simulink model "rpi_motor_cal"  (R2022b)
settings: Solver=FixedStepAuto  StartTime=0.0  StopTime=2  RelTol=1e-3  EnableMultiTasking=on
undefined symbols (not defined in the file or in its folder): A, b
libraries: raspberrypiBasiclib x6, robotmobilelib x1, raspberrypiIMUsensorslib x1, dspsigops x1
settings Model: Creator=sjohnson  LastModifiedBy=sjohnson
settings SolverCC: PositivePriorityOrder=on
settings OptimizationCC: EnhancedBackFolding=on  PassReuseOutputArgsAs=Individual arguments  ZeroExternalMemoryAtStartup=off  ZeroInternalMemoryAtStartup=off  MaxStackSize=64  OptimizeBlockOrder=speed  DifferentSizesBufferReuse=on  OptimizationCustomize=off  EfficientTunableParamExpr=on
settings DebuggingCC: ParameterTunabilityLossMsg=error
settings HardwareCC: ProdBitPerPointer=32  ProdBitPerSizeT=32  ProdBitPerPtrDiffT=32  ProdLargestAtomicInteger=Long  ProdLargestAtomicFloat=Double  ProdWordSize=32  ProdLongLongMode=on  ProdHWDeviceType=ARM Compatible->ARM Cortex  UseEmbeddedCoderFeatures=off  UseSimulinkCoderFeatures=off
settings RTWCC: Description=Embedded Coder  SystemTargetFile=ert.tlc  HardwareBoard=Raspberry Pi  TLCOptions="-aInlineSetEventsForThisBaseRateFcn=TLC_FALSE -aSuppressMultiTaskScheduler=TLC_FALSE  -aRateBasedStepFcn=0"  TemplateMakefile=ert_default_tmf  Toolchain=GNU GCC Embedded Linux  BuildConfiguration=Faster Runs
settings CodeAppCC: ForceParamTrailComments=on  IgnoreCustomStorageClasses=off  OperatorAnnotations=on  SimulinkDataObjDesc=on  SFDataObjDesc=on  InsertBlockDesc=on
settings ERTTargetCC: SupportNonInlinedSFcns=on  SupportVariableSizeSignals=on  ExtModeTransport=2  ExtModeStaticAlloc=on  ExtModeMexFile=ext_xcp  ExtModeIntrfLevel=Level2 - Open

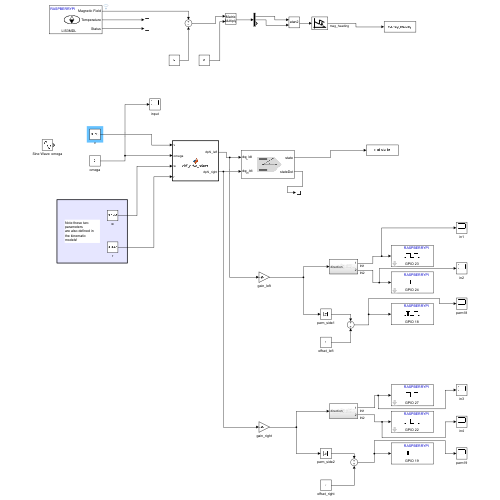
[thumbnail: Simulink's stored preview of the top-level diagram]
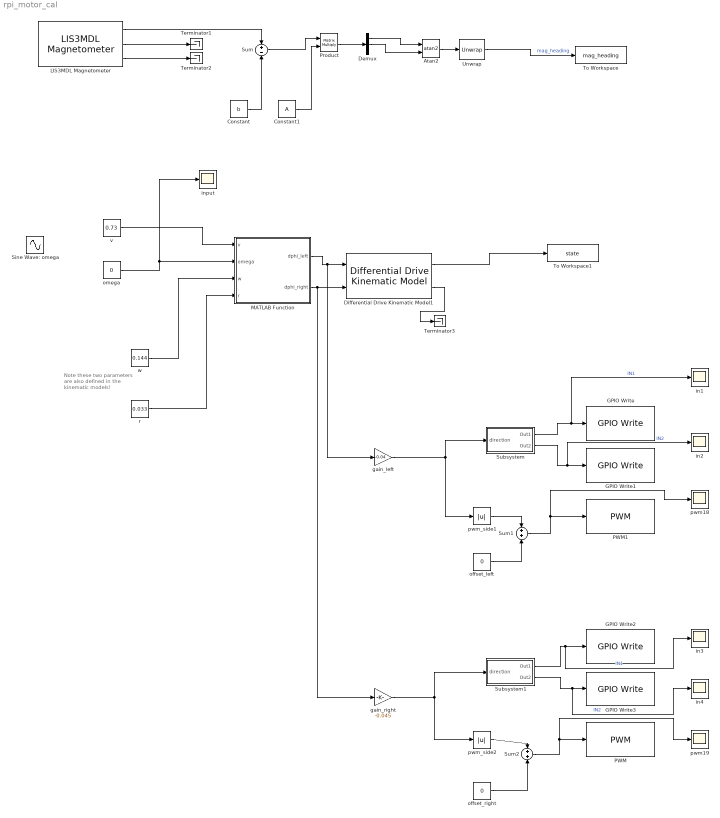
== system rpi_motor_cal ==
  note: Note these two parameters
      | are also defined in the kinematic
      | models!
  Atan2 : Trigonometry  Operator=atan2
  Constant : Constant  Value=b
  Constant1 : Constant  Value=A
  Demux : Demux  Outputs=3
  Differential Drive Kinematic Model1 : robotmobilelib/Differential Drive Kinematic Model  VehicleInputs=Wheel Speeds  WheelRadius=.033  WheelSpeedRange=[-inf inf]  TrackWidth=0.144  InitialState=[0; 0; 0]  SimulateUsing=Interpreted execution
  GPIO Write : raspberrypiBasiclib/GPIO Write  board=Pi 4 Model B  gpio=23  direction=Output  blockPlatform=Raspberry Pi
  GPIO Write1 : raspberrypiBasiclib/GPIO Write  board=Pi 4 Model B  gpio=24  direction=Output  blockPlatform=Raspberry Pi
  GPIO Write2 : raspberrypiBasiclib/GPIO Write  board=Pi 4 Model B  gpio=27  direction=Output  blockPlatform=Raspberry Pi
  GPIO Write3 : raspberrypiBasiclib/GPIO Write  board=Pi 4 Model B  gpio=22  direction=Output  blockPlatform=Raspberry Pi
  LIS3MDL Magnetometer : raspberrypiIMUsensorslib/LIS3MDL Magnetometer  I2CModule=1  I2CAddress=0x1E  IsActiveMagnetometer=on  IsActiveTemperature=on  IsStatus=on  SampleTime=-1  MagnetometerRange=+/- 400 uT  MagnetometerODR=40 Hz
  MATLAB Function : MATLAB Function  TreatAsAtomicUnit=on
  PWM : raspberrypiBasiclib/PWM  board=Pi 4 Model B  Pin_=19  Frequency=50  blockPlatform=Raspberry Pi
  PWM1 : raspberrypiBasiclib/PWM  board=Pi 4 Model B  Pin_=18  Frequency=50  blockPlatform=Raspberry Pi
  Product : Product  Multiplication=Matrix(*)
  Sine Wave: omega : Sin  Amplitude=0.1  Frequency=0.1  SampleTime=0
  Subsystem : Subsystem
  Subsystem1 : Subsystem
  Sum : Sum  Inputs=+-
  Sum1 : Sum
  Sum2 : Sum
  Terminator1 : Terminator
  Terminator2 : Terminator
  Terminator3 : Terminator
  To Workspace : ToWorkspace  VariableName=mag_heading  SaveFormat=Structure With Time  SampleTime=-1
  To Workspace1 : ToWorkspace  VariableName=state  SaveFormat=Structure With Time  SampleTime=-1
  Unwrap : dspsigops/Unwrap  tol=pi  InputProcessing=Columns as channels (frame based)  running=off
  gain_left : Gain  Gain=-0.04
  gain_right : Gain  Gain=-0.045
  in{1..4} (4 alike) : Scope
  input : Scope
  offset_left : Constant  Value=0
  offset_right : Constant  Value=0
  omega : Constant  Value=0
  pwm18 : Scope
  pwm19 : Scope
  pwm_side1 : Abs  SaturateOnIntegerOverflow=off
  pwm_side2 : Abs  SaturateOnIntegerOverflow=off
  r : Constant  Value=0.033
  v : Constant  Value=0.73
  w : Constant  Value=0.144
  wires:
  LIS3MDL Magnetometer/2 -> Terminator1/1
  Product/1 -> Demux/1
  Constant1/1 -> Product/2
  LIS3MDL Magnetometer/1 -> Sum/1
  Sum/1 -> Product/1
  Atan2/1 -> Unwrap/1
  Demux/1 -> Atan2/1
  LIS3MDL Magnetometer/3 -> Terminator2/1
  Constant/1 -> Sum/2
  Demux/2 -> Atan2/2
  v/1 -> MATLAB Function/1(v)
  MATLAB Function/1(dphi_left) -> gain_left/1, Differential Drive Kinematic Model1/1
  omega/1 -> input/1, MATLAB Function/2(omega)
  Differential Drive Kinematic Model1/2 -> Terminator3/1
  w/1 -> MATLAB Function/3(w)
  r/1 -> MATLAB Function/4(r)
  Subsystem/1(Out1) -> in1/1, GPIO Write/1  "IN1"
  gain_left/1 -> Subsystem/1(direction), pwm_side1/1
  Subsystem/2(Out2) -> in2/1, GPIO Write1/1  "IN2"
  Sum1/1 -> pwm18/1, PWM1/1
  Sum2/1 -> PWM/1, pwm19/1
  gain_right/1 -> Subsystem1/1(direction), pwm_side2/1
  Subsystem1/1(Out1) -> in3/1, GPIO Write2/1  "IN1"
  Subsystem1/2(Out2) -> in4/1, GPIO Write3/1  "IN2"
  offset_left/1 -> Sum1/2
  offset_right/1 -> Sum2/2
  MATLAB Function/2(dphi_right) -> gain_right/1, Differential Drive Kinematic Model1/2
  Unwrap/1 -> To Workspace/1  "mag_heading"
  Differential Drive Kinematic Model1/1 -> To Workspace1/1
  pwm_side1/1 -> Sum1/1
  pwm_side2/1 -> Sum2/1

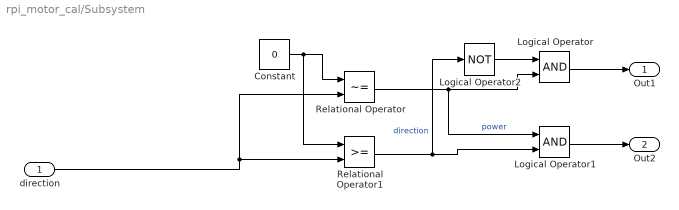
== system rpi_motor_cal/Subsystem ==
  direction : Inport
  Constant : Constant  Value=0
  Logical Operator : Logic  AllPortsSameDT=off  OutDataTypeStr=boolean
  Logical Operator1 : Logic  AllPortsSameDT=off  OutDataTypeStr=boolean
  Logical Operator2 : Logic  Operator=NOT  Inputs=1  AllPortsSameDT=off  OutDataTypeStr=boolean
  Relational Operator : RelationalOperator  Operator=~=  OutDataTypeStr=boolean  RndMeth=Simplest  InputSameDT=off
  Relational Operator1 : RelationalOperator  OutDataTypeStr=boolean  RndMeth=Simplest  InputSameDT=off
  Out1 : Outport
  Out2 : Outport  Port=2
  wires:
  Logical Operator/1 -> Out1/1
  Relational Operator1/1 -> Logical Operator2/1, Logical Operator1/2  "direction"
  Logical Operator1/1 -> Out2/1
  Logical Operator2/1 -> Logical Operator/1
  direction/1 -> Relational Operator/2, Relational Operator1/2
  Constant/1 -> Relational Operator1/1, Relational Operator/1
  Relational Operator/1 -> Logical Operator1/1, Logical Operator/2  "power"

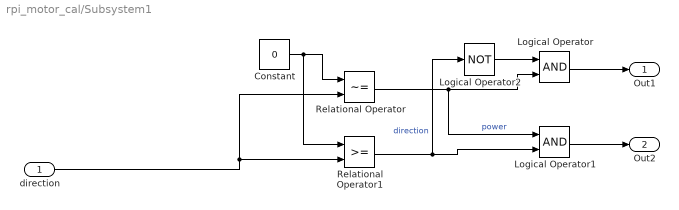
== system rpi_motor_cal/Subsystem1 ==
  direction : Inport
  Constant : Constant  Value=0
  Logical Operator : Logic  AllPortsSameDT=off  OutDataTypeStr=boolean
  Logical Operator1 : Logic  AllPortsSameDT=off  OutDataTypeStr=boolean
  Logical Operator2 : Logic  Operator=NOT  Inputs=1  AllPortsSameDT=off  OutDataTypeStr=boolean
  Relational Operator : RelationalOperator  Operator=~=  OutDataTypeStr=boolean  RndMeth=Simplest  InputSameDT=off
  Relational Operator1 : RelationalOperator  OutDataTypeStr=boolean  RndMeth=Simplest  InputSameDT=off
  Out1 : Outport
  Out2 : Outport  Port=2
  wires:
  Logical Operator/1 -> Out1/1
  Relational Operator1/1 -> Logical Operator2/1, Logical Operator1/2  "direction"
  Logical Operator1/1 -> Out2/1
  Logical Operator2/1 -> Logical Operator/1
  direction/1 -> Relational Operator/2, Relational Operator1/2
  Constant/1 -> Relational Operator1/1, Relational Operator/1
  Relational Operator/1 -> Logical Operator1/1, Logical Operator/2  "power"

== matlab function rpi_motor_cal/MATLAB Function ==
  data: v input; dphi_left output; omega input; w input; r input; dphi_right output
function [dphi_left, dphi_right] = diff_drive_xform(v, omega, w, r)

c1 = w/(2*r);
c2 = 2/w;

dphi_left = c1 * ( c2*v - omega );
dphi_right = c1 * ( c2*v + omega );
